simulink model "HP_Butter_2nd"  (R2020a)
settings: Solver=FixedStepDiscrete  StartTime=0.0  StopTime=840000  RelTol=1e-3
settings Model: FPTRunName=FPA_Reference  PacingRate=40  Creator=BuccelliLab  LastModifiedBy=diflo
settings SolverCC: AutoInsertRateTranBlk=on  MinimalZcImpactIntegration=on
settings DataIOCC: LimitDataPoints=on  SaveOutput=off  SaveTime=off  ReturnWorkspaceOutputs=off
settings OptimizationCC: BlockReduction=off  ConditionallyExecuteInputs=off  DefaultParameterBehavior=Inlined  LifeSpan=inf
settings DebuggingCC: SignalRangeChecking=warning  ReadBeforeWriteMsg=DisableAll  WriteAfterWriteMsg=DisableAll  WriteAfterReadMsg=DisableAll  AlgebraicLoopMsg=error  MultiTaskDSMMsg=none  SingleTaskRateTransMsg=error  ParameterDowncastMsg=warning  ParameterOverflowMsg=warning  AllowSymbolicDim=off  StrictBusMsg=ErrorOnBusTreatedAsVector  SFUnexpectedBacktrackingDiag=warning  SFNoUnconditionalDefaultTransitionDiag=warning  SFExecutionAtInitializationDiag=none  ArithmeticOperatorsInVariantConditions=warning
settings HardwareCC: ProdBitPerPointer=32  ProdBitPerSizeT=32  ProdBitPerPtrDiffT=32  ProdLargestAtomicFloat=None  ProdIntDivRoundTo=Undefined  ProdEndianess=Unspecified  ProdWordSize=32  ProdHWDeviceType=ASIC/FPGA->ASIC/FPGA  TargetBitPerPointer=64  TargetBitPerSizeT=64  TargetBitPerPtrDiffT=64  TargetLongLongMode=on  TargetIntDivRoundTo=Zero  TargetEndianess=LittleEndian  TargetWordSize=64  TargetHWDeviceType=Custom Processor->MATLAB Host Computer  ProdEqTarget=off
settings ModelReferenceCC: UpdateModelReferenceTargets=IfOutOfDate
settings SFSimCC: SFSimEcho=off  SimUseLocalCustomCode=off  CustomCodeUndefinedFunction=UseInterfaceOnly
settings RTWCC: RTWUseLocalCustomCode=off
settings CodeAppCC: StateflowObjectComments=on
settings GRTTargetCC: TargetLangStandard=C89/C90 (ANSI)
settings ConfigComp: CovScope=ReferencedModels  CovMetricSettings=dw  CovHtmlReporting=on  CovSaveCumulativeToWorkspaceVar=on  CovSaveSingleToWorkspaceVar=on  CovExternalEMLEnable=off  CovSFcnEnable=off

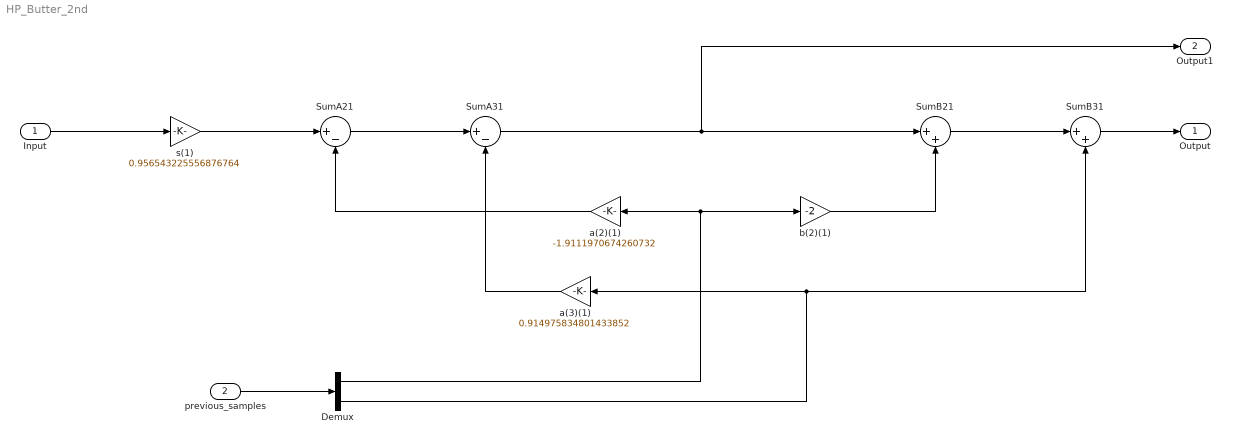
== system HP_Butter_2nd ==
  Input : Inport  OutDataTypeStr=fixdt(1,32,15)  PortDimensions=1  SampleTime=[1,0]
  previous_samples : Inport  Port=2  OutDataTypeStr=fixdt(1,32,7)  PortDimensions=2  SampleTime=[1,0]
  Demux : Demux  Outputs=2
  SumA21 : Sum  Inputs=|+-  AccumDataTypeStr=fixdt(1,32,6)  OutDataTypeStr=fixdt(1,32,6)  RndMeth=Nearest  SaturateOnIntegerOverflow=on
  SumA31 : Sum  Inputs=|+-  AccumDataTypeStr=fixdt(1,32,6)  OutDataTypeStr=fixdt(1,32,7)  RndMeth=Nearest  SaturateOnIntegerOverflow=on
  SumB21 : Sum  Inputs=|++  AccumDataTypeStr=fixdt(1,32,6)  OutDataTypeStr=fixdt(1,32,7)  RndMeth=Nearest  SaturateOnIntegerOverflow=on
  SumB31 : Sum  Inputs=|++  AccumDataTypeStr=fixdt(1,32,7)  OutDataTypeStr=fixdt(1,32,15)  RndMeth=Nearest  SaturateOnIntegerOverflow=on
  a(2)(1) : Gain  Gain=-1.9111970674260732  ParamDataTypeStr=fixdt(1,32,30)  OutDataTypeStr=fixdt(1,32,6)  RndMeth=Nearest  SaturateOnIntegerOverflow=on
  a(3)(1) : Gain  Gain=0.914975834801433852  ParamDataTypeStr=fixdt(0,32,32)  OutDataTypeStr=fixdt(1,32,8)  RndMeth=Nearest  SaturateOnIntegerOverflow=on
  b(2)(1) : Gain  Gain=-2  ParamDataTypeStr=fixdt(1,32,30)  OutDataTypeStr=fixdt(1,32,6)  RndMeth=Nearest  SaturateOnIntegerOverflow=on
  s(1) : Gain  Gain=0.956543225556876764  ParamDataTypeStr=fixdt(0,32,32)  OutDataTypeStr=fixdt(1,32,16)  RndMeth=Nearest  SaturateOnIntegerOverflow=on
  Output : Outport  OutDataTypeStr=fixdt(1,32,15)  PortDimensions=1  SampleTime=[1,0]
  Output1 : Outport  Port=2  OutDataTypeStr=fixdt(1,32,7)  PortDimensions=1  SampleTime=[1,0]
  wires:
  previous_samples/1 -> Demux/1
  Input/1 -> s(1)/1
  SumB31/1 -> Output/1
  Demux/1 -> a(2)(1)/1, b(2)(1)/1
  SumA21/1 -> SumA31/1
  a(3)(1)/1 -> SumA31/2
  SumA31/1 -> Output1/1, SumB21/1
  b(2)(1)/1 -> SumB21/2
  Demux/2 -> a(3)(1)/1, SumB31/2
  SumB21/1 -> SumB31/1
  s(1)/1 -> SumA21/1
  a(2)(1)/1 -> SumA21/2
